simulink model "HybridCarModel"  (R2023a)
settings: Solver=VariableStepAuto  StartTime=0.0  StopTime=10.0  RelTol=1e-3
model workspace (MAT data in the model file):
  Aeff : Simulink.Parameter (value not decoded)
  Af : Simulink.Parameter (value not decoded)
  BattCapInit : Simulink.Parameter (value not decoded)
  BattChargeMax : Simulink.Parameter (value not decoded)
  BattTempBp : Simulink.Parameter (value not decoded)
  Bx : Simulink.Parameter (value not decoded)
  CapLUTBp : Simulink.Parameter (value not decoded)
  CapSOCBp : Simulink.Parameter (value not decoded)
  CatLightOffTime : Simulink.Parameter (value not decoded)
  Cd : Simulink.Parameter (value not decoded)
  Cl : Simulink.Parameter (value not decoded)
  Cpm : Simulink.Parameter (value not decoded)
  Cps : Simulink.Parameter (value not decoded)
  CrankSpeed : Simulink.Parameter (value not decoded)
  Cx : Simulink.Parameter (value not decoded)
  Dx : Simulink.Parameter (value not decoded)
  Em : Simulink.Parameter (value not decoded)
  EngRevLim : Simulink.Parameter (value not decoded)
  EngStopStartEnable : Simulink.Parameter (value not decoded)
  EngStopTime : Simulink.Parameter (value not decoded)
  Ex : Simulink.Parameter (value not decoded)
  FZMAX : Simulink.Parameter (value not decoded)
  FZMIN : Simulink.Parameter (value not decoded)
  Fc : Simulink.Parameter (value not decoded)
  FsbF : Simulink.Parameter (value not decoded)
  FsbR : Simulink.Parameter (value not decoded)
  FskF : Simulink.Parameter (value not decoded)
  FskR : Simulink.Parameter (value not decoded)
  G : Simulink.Parameter (value not decoded)
  G_o : Simulink.Parameter (value not decoded)
  Iyy : Simulink.Parameter (value not decoded)
  Iyy_Whl : Simulink.Parameter (value not decoded)
  J : Simulink.Parameter (value not decoded)
  J1 : Simulink.Parameter (value not decoded)
  J2 : Simulink.Parameter (value not decoded)
  Jd : Simulink.Parameter (value not decoded)
  Ji : Simulink.Parameter (value not decoded)
  Jin : Simulink.Parameter (value not decoded)
  Jin_Cltch : Simulink.Parameter (value not decoded)
  Jin_Cltch2 : Simulink.Parameter (value not decoded)
  Jout : Simulink.Parameter (value not decoded)
  Jout_Cltch : Simulink.Parameter (value not decoded)
  Jout_Cltch2 : Simulink.Parameter (value not decoded)
  Jt : Simulink.Parameter (value not decoded)
  Jw1 : Simulink.Parameter (value not decoded)
  Jw2 : Simulink.Parameter (value not decoded)
  K_c : Simulink.Parameter (value not decoded)
  Lrel : Simulink.Parameter (value not decoded)
  Mass : Simulink.Parameter (value not decoded)
  N : Simulink.Parameter (value not decoded)
  NCyl : Simulink.Parameter (value not decoded)
  NF : Simulink.Parameter (value not decoded)
  NR : Simulink.Parameter (value not decoded)
  N_P4 : Simulink.Parameter (value not decoded)
  N_idle : Simulink.Parameter (value not decoded)
  Ndiff : Simulink.Parameter (value not decoded)
  Ndiff_P4 : Simulink.Parameter (value not decoded)
  Ndisk : Simulink.Parameter (value not decoded)
  Ndisks : Simulink.Parameter (value not decoded)
  Np : Simulink.Parameter (value not decoded)
  Ns : Simulink.Parameter (value not decoded)
  Pabs : Simulink.Parameter (value not decoded)
  Plimit : Simulink.Parameter (value not decoded)
  Press : Simulink.Parameter (value not decoded)
  Pstd : Simulink.Parameter (value not decoded)
  RInt : Simulink.Parameter (value not decoded)
  Rair : Simulink.Parameter (value not decoded)
  Re : Simulink.Parameter (value not decoded)
  Reff : Simulink.Parameter (value not decoded)
  Reff_LSD : Simulink.Parameter (value not decoded)
  Rm : Simulink.Parameter (value not decoded)
  Sinj : Simulink.Parameter (value not decoded)
  T : Simulink.Parameter (value not decoded)
  T_eff_bp : Simulink.Parameter (value not decoded)
  T_t : Simulink.Parameter (value not decoded)
  Tc : Simulink.Parameter (value not decoded)
  Temp_bpts : Simulink.Parameter (value not decoded)
  Trq_bpts : Simulink.Parameter (value not decoded)
  Ts : Simulink.Parameter (value not decoded)
  Tstd : Simulink.Parameter (value not decoded)
  UNLOADED_RADIUS : Simulink.Parameter (value not decoded)
  VXLOW : Simulink.Parameter (value not decoded)
  Vd : Simulink.Parameter (value not decoded)
  Vinit : Simulink.Parameter (value not decoded)
  aMy : Simulink.Parameter (value not decoded)
  a_CG : Simulink.Parameter (value not decoded)
  afr_stoich : Simulink.Parameter (value not decoded)
  alphaMy : Simulink.Parameter (value not decoded)
  b : Simulink.Parameter (value not decoded)
  b1 : Simulink.Parameter (value not decoded)
  b1_g : Simulink.Parameter (value not decoded)
  b2 : Simulink.Parameter (value not decoded)
  b2_g : Simulink.Parameter (value not decoded)
  bMy : Simulink.Parameter (value not decoded)
  b_CG : Simulink.Parameter (value not decoded)
  b_J : Simulink.Parameter (value not decoded)
  bd : Simulink.Parameter (value not decoded)
  betaMy : Simulink.Parameter (value not decoded)
  bi : Simulink.Parameter (value not decoded)
  bin : Simulink.Parameter (value not decoded)
  bin_Cltch : Simulink.Parameter (value not decoded)
  bout : Simulink.Parameter (value not decoded)
  bout_Cltch : Simulink.Parameter (value not decoded)
  br : Simulink.Parameter (value not decoded)
  bt : Simulink.Parameter (value not decoded)
  bw1 : Simulink.Parameter (value not decoded)
  bw2 : Simulink.Parameter (value not decoded)
  cMy : Simulink.Parameter (value not decoded)
  calEngVar : object (value not decoded)
  disk_abore : Simulink.Parameter (value not decoded)
  domega_o : Simulink.Parameter (value not decoded)
  dw : Simulink.Parameter (value not decoded)
  dzdotsF : Simulink.Parameter (value not decoded)
  dzdotsR : Simulink.Parameter (value not decoded)
  dzsF : Simulink.Parameter (value not decoded)
  dzsR : Simulink.Parameter (value not decoded)
  eff : Simulink.Parameter (value not decoded)
  efficiency_table : Simulink.Parameter (value not decoded)
  eta : Simulink.Parameter (value not decoded)
  eta_diff : Simulink.Parameter (value not decoded)
  eta_tbl : Simulink.Parameter (value not decoded)
  f_cp_ld_bpt : Simulink.Parameter (value not decoded)
  f_cp_n_bpt : Simulink.Parameter (value not decoded)
  f_del_sa_bpt : Simulink.Parameter (value not decoded)
  f_ecp : Simulink.Parameter (value not decoded)
  f_egr_areapct_cmd : Simulink.Parameter (value not decoded)
  f_egr_areapct_nrmlzdflow_bpt : Simulink.Parameter (value not decoded)
  f_egr_areapct_pr_bpt : Simulink.Parameter (value not decoded)
  f_egr_max_stdflow : Simulink.Parameter (value not decoded)
  f_egr_stdflow : Simulink.Parameter (value not decoded)
  f_egr_stdflow_egrap_bpt : Simulink.Parameter (value not decoded)
  f_egr_stdflow_pr_bpt : Simulink.Parameter (value not decoded)
  f_egrpct_cmd : Simulink.Parameter (value not decoded)
  f_egrpct_ld_bpt : Simulink.Parameter (value not decoded)
  f_egrpct_n_bpt : Simulink.Parameter (value not decoded)
  f_fric_temp_bpt : Simulink.Parameter (value not decoded)
  f_fric_temp_mod : Simulink.Parameter (value not decoded)
  f_icp : Simulink.Parameter (value not decoded)
  f_intksys_stdflow_bpt : Simulink.Parameter (value not decoded)
  f_intksys_stdflow_pr : Simulink.Parameter (value not decoded)
  f_lamcmd : Simulink.Parameter (value not decoded)
  f_lamcmd_ld_bpt : Simulink.Parameter (value not decoded)
  f_lamcmd_n_bpt : Simulink.Parameter (value not decoded)
  f_lcmd : Simulink.Parameter (value not decoded)
  f_lcmd_n_bpt : Simulink.Parameter (value not decoded)
  f_lcmd_tq_bpt : Simulink.Parameter (value not decoded)
  f_m_lam : Simulink.Parameter (value not decoded)
  f_m_lam_bpt : Simulink.Parameter (value not decoded)
  f_m_sa : Simulink.Parameter (value not decoded)
  f_mdot_air_corr : Simulink.Parameter (value not decoded)
  f_mdot_air_corr_ld_bpt : Simulink.Parameter (value not decoded)
  f_mdot_air_n_bpt : Simulink.Parameter (value not decoded)
  f_mdot_intk : Simulink.Parameter (value not decoded)
  f_mdot_intk_ecp_bpt : Simulink.Parameter (value not decoded)
  f_mdot_trpd_bpt : Simulink.Parameter (value not decoded)
  f_nv : Simulink.Parameter (value not decoded)
  f_nv_n_bpt : Simulink.Parameter (value not decoded)
  f_nv_prs_bpt : Simulink.Parameter (value not decoded)
  f_sa : Simulink.Parameter (value not decoded)
  f_sa_ld_bpt : Simulink.Parameter (value not decoded)
  f_sa_n_bpt : Simulink.Parameter (value not decoded)
  f_sa_opt : Simulink.Parameter (value not decoded)
  f_startup_ect_bpt : Simulink.Parameter (value not decoded)
  f_startup_lambda_delta : Simulink.Parameter (value not decoded)
  f_startup_lambda_delta_timecnst : Simulink.Parameter (value not decoded)
  f_t_exh : Simulink.Parameter (value not decoded)
  f_t_exh_l_bpt : Simulink.Parameter (value not decoded)
  f_t_exh_n_bpt : Simulink.Parameter (value not decoded)
  f_tap : Simulink.Parameter (value not decoded)
  f_tap_ld_bpt : Simulink.Parameter (value not decoded)
  f_tap_n_bpt : Simulink.Parameter (value not decoded)
  f_tm_corr : Simulink.Parameter (value not decoded)
  f_tm_corr_n_bpt : Simulink.Parameter (value not decoded)
  f_tm_corr_nd_bpt : Simulink.Parameter (value not decoded)
  f_tpp : Simulink.Parameter (value not decoded)
  f_tpp_tap_bpt : Simulink.Parameter (value not decoded)
  f_tq_fric : Simulink.Parameter (value not decoded)
  f_tq_inr : Simulink.Parameter (value not decoded)
  f_tq_inr_l_bpt : Simulink.Parameter (value not decoded)
  f_tq_inr_n_bpt : Simulink.Parameter (value not decoded)
  f_tq_nl : Simulink.Parameter (value not decoded)
  f_tq_nl_l_bpt : Simulink.Parameter (value not decoded)
  f_tq_nl_n_bpt : Simulink.Parameter (value not decoded)
  f_tq_pump : Simulink.Parameter (value not decoded)
  f_vivc : Simulink.Parameter (value not decoded)
  f_vivc_icp_bpt : Simulink.Parameter (value not decoded)
  f_wap : Simulink.Parameter (value not decoded)
  f_wap_ld_bpt : Simulink.Parameter (value not decoded)
  f_wap_n_bpt : Simulink.Parameter (value not decoded)
  g : Simulink.Parameter (value not decoded)
  grEff : Simulink.Parameter (value not decoded)
  h : Simulink.Parameter (value not decoded)
  k : Simulink.Parameter (value not decoded)
  k1 : Simulink.Parameter (value not decoded)
  k2 : Simulink.Parameter (value not decoded)
  kappamax : Simulink.Parameter (value not decoded)
  lam_x : Simulink.Parameter (value not decoded)
  mu_kinetic : Simulink.Parameter (value not decoded)
  mu_static : Simulink.Parameter (value not decoded)
  muc : Simulink.Parameter (value not decoded)
  muk : Simulink.Parameter (value not decoded)
  mus : Simulink.Parameter (value not decoded)
  num_pads : Simulink.Parameter (value not decoded)
  omega1_c : Simulink.Parameter (value not decoded)
  omega2_c : Simulink.Parameter (value not decoded)
  omega_bpts : Simulink.Parameter (value not decoded)
  omega_c : Simulink.Parameter (value not decoded)
  omega_o : Simulink.Parameter (value not decoded)
  omega_o_J : Simulink.Parameter (value not decoded)
  omegai_o : Simulink.Parameter (value not decoded)
  omegain_o : Simulink.Parameter (value not decoded)
  omegal : Simulink.Parameter (value not decoded)
  omegao : Simulink.Parameter (value not decoded)
  omegaout_o : Simulink.Parameter (value not decoded)
  omegat_o : Simulink.Parameter (value not decoded)
  omegau : Simulink.Parameter (value not decoded)
  omegaw1o : Simulink.Parameter (value not decoded)
  omegaw2o : Simulink.Parameter (value not decoded)
  phi : Simulink.Parameter (value not decoded)
  philu : Simulink.Parameter (value not decoded)
  power_max : Simulink.Parameter (value not decoded)
  press : Simulink.Parameter (value not decoded)
  psi : Simulink.Parameter (value not decoded)
  q_o : Simulink.Parameter (value not decoded)
  tauC : Simulink.Parameter (value not decoded)
  tauC_1 : Simulink.Parameter (value not decoded)
  tauC_LSD : Simulink.Parameter (value not decoded)
  tauTC : Simulink.Parameter (value not decoded)
  tau_egr : Simulink.Parameter (value not decoded)
  tau_s : Simulink.Parameter (value not decoded)
  tc : Simulink.Parameter (value not decoded)
  theta_o : Simulink.Parameter (value not decoded)
  theta_o_Veh : Simulink.Parameter (value not decoded)
  torque_max : Simulink.Parameter (value not decoded)
  ts : Simulink.Parameter (value not decoded)
  w1_o : Simulink.Parameter (value not decoded)
  w_eff_bp : Simulink.Parameter (value not decoded)
  wc : Simulink.Parameter (value not decoded)
  win_o : Simulink.Parameter (value not decoded)
  wout_o : Simulink.Parameter (value not decoded)
  x_o : Simulink.Parameter (value not decoded)
  xdot_o : Simulink.Parameter (value not decoded)
  z_o : Simulink.Parameter (value not decoded)
  zdot_o : Simulink.Parameter (value not decoded)
  zeta : Simulink.Parameter (value not decoded)
symbols that are objects in the model workspace (value not decoded): b, b_CG, BattCapInit, BattChargeMax, CapLUTBp, Em, g, k, Mass, N, Ns, T, w_eff_bp
undefined symbols (not defined in the file or in its folder): Lock, up
libraries: autolibpowerinfoutils x5, autolibsharedcoupling x4, autolibshared x3, autolibutils x2, autolibshareddiff x2, autolibsharedmappedengines x1, autolibdcdc x1, autolibdatasheetbattery x1, autolibmappedmotor x1, autolibsharedtransfixedgear x1, autolibtrqconv x1
(part 3 of 3)

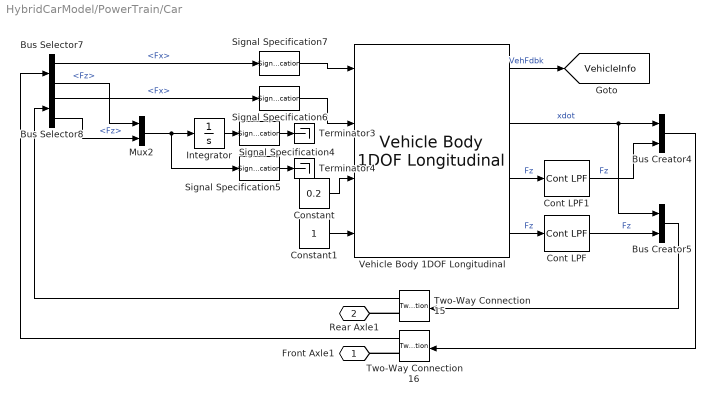
== system HybridCarModel/PowerTrain/Car ==
  Bus Creator4 : BusCreator  Inputs=2
  Bus Creator5 : BusCreator  Inputs=2
  Bus Selector7 : BusSelector  OutputSignals=Fx,Fz
  Bus Selector8 : BusSelector  OutputSignals=Fx,Fz
  Constant : Constant  Value=0.2
  Constant1 : Constant
  Cont LPF : autolibutils/Cont LPF  wc=wc  AbsoluteTolerance=auto  aMode=aMode
  Cont LPF1 : autolibutils/Cont LPF  wc=wc  AbsoluteTolerance=auto  aMode=aMode
  Integrator : Integrator
  Mux2 : Mux  Inputs=2
  Signal Specification4 : SignalSpecification  Unit=m
  Signal Specification5 : SignalSpecification  Unit=m/s
  Signal Specification6 : SignalSpecification  Unit=N
  Signal Specification7 : SignalSpecification  Unit=N
  Terminator3 : Terminator
  Terminator4 : Terminator
  Two-Way Connection15 : TwoWayConnection
  Two-Way Connection16 : TwoWayConnection
  Vehicle Body 1DOF Longitudinal : autolibshared/Vehicle Body 1DOF Longitudinal  VariantControl=SL  extFMode=off  extMMode=off  extTamb=off  wind3D=off  aMode=1  NF=NF  NR=NR  m=Mass  a=a_CG  b=b_CG  h=h  Cd=Cd  Cl=0  Cpm=0  Af=Af  x_o=x_o  xdot_o=xdot_o  Pabs=Pabs  T=T  g=g
      settings: LibrarySourceBlock=autolibvehdynlong/Vehicle Body 1DOF Longitudinal
  Front Axle1 : PMIOPort  Side=Left
  Rear Axle1 : PMIOPort  Port=2  Side=Left
  tag scope: VehicleInfo=global
  wires:
  Mux2/1 -> Signal Specification5/1, Integrator/1
  Vehicle Body 1DOF Longitudinal/2 -> Bus Creator4/1, Bus Creator5/1  "xdot"
  Bus Selector8/2 -> Mux2/2  "<Fz>"
  Bus Selector8/1 -> Signal Specification6/1  "<Fx>"
  Cont LPF1/1 -> Bus Creator4/2  "Fz"
  Bus Selector7/2 -> Mux2/1  "<Fz>"
  Signal Specification6/1 -> Vehicle Body 1DOF Longitudinal/2
  Two-Way Connection15/1 -> Bus Selector8/1
  Integrator/1 -> Signal Specification4/1
  Vehicle Body 1DOF Longitudinal/3 -> Cont LPF1/1  "Fz"
  Bus Creator5/1 -> Two-Way Connection15/1
  Signal Specification7/1 -> Vehicle Body 1DOF Longitudinal/1
  Vehicle Body 1DOF Longitudinal/1 -> [VehicleInfo]  "VehFdbk"
  Cont LPF/1 -> Bus Creator5/2  "Fz"
  Bus Creator4/1 -> Two-Way Connection16/1
  Bus Selector7/1 -> Signal Specification7/1  "<Fx>"
  Two-Way Connection16/1 -> Bus Selector7/1
  Signal Specification5/1 -> Terminator4/1
  Signal Specification4/1 -> Terminator3/1
  Vehicle Body 1DOF Longitudinal/4 -> Cont LPF/1  "Fz"
  Constant/1 -> Vehicle Body 1DOF Longitudinal/3
  Constant1/1 -> Vehicle Body 1DOF Longitudinal/4
  connections:
  Two-Way Connection16/RConn1 -- Front Axle1/RConn1
  Two-Way Connection15/RConn1 -- Rear Axle1/RConn1

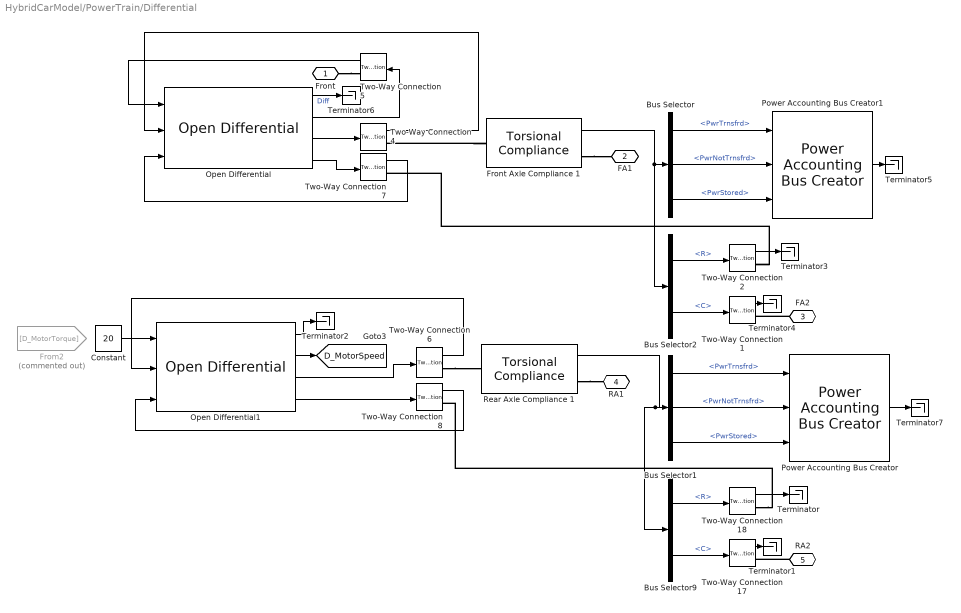
== system HybridCarModel/PowerTrain/Differential ==
  Bus Selector : BusSelector  OutputSignals=PwrInfo.PwrTrnsfrd,PwrInfo.PwrNotTrnsfrd,PwrInfo.PwrStored
  Bus Selector1 : BusSelector  OutputSignals=PwrInfo.PwrTrnsfrd,PwrInfo.PwrNotTrnsfrd,PwrInfo.PwrStored
  Bus Selector2 : BusSelector  OutputSignals=Trq.R,Trq.C
  Bus Selector9 : BusSelector  OutputSignals=Trq.R,Trq.C
  Constant : Constant  Value=20
  From2 : From  Commented=on  GotoTag=D_MotorTorque
  Front Axle Compliance 1 : autolibsharedcoupling/Torsional Compliance  port_config=Two-way connection  extInfo=on  k=k  b=b  theta_o=theta_o  domega_o=domega_o  omega_c=omega_c  blkID=0  aMode=1
  Open Differential : autolibshareddiff/Open Differential  DiffEffModelPopup=Constant  InterpMethod=Linear point-slope  extTamb=off  shaftSwitchMask=To the left of center-line  Ndiff=Ndiff  Jd=Jd  bd=bd  Jw1=Jw1  bw1=bw1  Jw2=Jw2  bw2=bw2  omegaw1o=omegaw1o  omegaw2o=omegaw2o  eta=eta_diff  eta_tbl=reshape([0.64 0.76 0.8 0.81 0.83 0.84 0.84 0.56 0.73 0.78 0.8 0.83 0.84 0.84 0.54 0.71 0.77 0.8 0.82 0.84 0.84 0.53 0.71 0.77 0.8 0.83 0.84 0.84 0.51 0.71 0.77 0.8 0.83 0.84 0.85 0.52 0.7 0.77 0.8 0.83 0.84 0.85 0.51 0.71 0.76 0.79 0.83 0.84 0.85 0.5 0.69 0.76 0.79 0.82 0.84 0.85 0.45 0.68 0.75 0.78 0.82 0.84 0.85 0.43 0.67 0.74 0.78 0.81 0.83 0.84 0.38 0.63 0.71 0.75 0.8 0.82 0.83 0.81 0.86 0.88 0.89 0.89 0.89 0.9 0.77 0.85 0.87 0.88 0.89 0.9 0.9 0.72 0.82 0.86 0.87 0.88 0.89 0.9 0.68 0.8 0.84 0.86 0.88 0.89 0.89 0.67 0.8 0.84 0.86 0.88 0.89 0.9 0.67 0.8 0.84 0.86 0.88 0.89 0.9 0.65 0.8 0.84 0.86 0.88 0.89 0.9 0.64 0.79 0.83 0.86 0.88 0.89 0.9 0.63 0.78 0.83 0.86 0.88 0.89 0.9 0.59 0.76 0.82 0.85 0.87 0.89 0.9 0.53 0.73 0.8 0.83 0.86 0.88 0.89], 7, 11, 2)  Trq_bpts=[25, 50, 75, 100, 150, 200, 250]  omega_bpts=[52.4 78.5 105 131 157 183 209 262 314 419 524]  Temp_bpts=[290 358]  Tamb=297.15  maxAbsSpd=5e3  aMode=1
      settings: LibrarySourceBlock=autolibdiff/Open Differential
  Open Differential1 : autolibshareddiff/Open Differential  DiffEffModelPopup=Constant  InterpMethod=Linear point-slope  extTamb=off  shaftSwitchMask=To the left of center-line  Ndiff=Ndiff_P4  Jd=Jd  bd=bd  Jw1=Jw1  bw1=bw1  Jw2=Jw2  bw2=bw2  omegaw1o=omegaw1o  omegaw2o=omegaw2o  eta=eta_diff  eta_tbl=reshape([0.64 0.76 0.8 0.81 0.83 0.84 0.84 0.56 0.73 0.78 0.8 0.83 0.84 0.84 0.54 0.71 0.77 0.8 0.82 0.84 0.84 0.53 0.71 0.77 0.8 0.83 0.84 0.84 0.51 0.71 0.77 0.8 0.83 0.84 0.85 0.52 0.7 0.77 0.8 0.83 0.84 0.85 0.51 0.71 0.76 0.79 0.83 0.84 0.85 0.5 0.69 0.76 0.79 0.82 0.84 0.85 0.45 0.68 0.75 0.78 0.82 0.84 0.85 0.43 0.67 0.74 0.78 0.81 0.83 0.84 0.38 0.63 0.71 0.75 0.8 0.82 0.83 0.81 0.86 0.88 0.89 0.89 0.89 0.9 0.77 0.85 0.87 0.88 0.89 0.9 0.9 0.72 0.82 0.86 0.87 0.88 0.89 0.9 0.68 0.8 0.84 0.86 0.88 0.89 0.89 0.67 0.8 0.84 0.86 0.88 0.89 0.9 0.67 0.8 0.84 0.86 0.88 0.89 0.9 0.65 0.8 0.84 0.86 0.88 0.89 0.9 0.64 0.79 0.83 0.86 0.88 0.89 0.9 0.63 0.78 0.83 0.86 0.88 0.89 0.9 0.59 0.76 0.82 0.85 0.87 0.89 0.9 0.53 0.73 0.8 0.83 0.86 0.88 0.89], 7, 11, 2)  Trq_bpts=[25, 50, 75, 100, 150, 200, 250]  omega_bpts=[52.4 78.5 105 131 157 183 209 262 314 419 524]  Temp_bpts=[290 358]  Tamb=297.15  maxAbsSpd=5e3  aMode=1
      settings: LibrarySourceBlock=autolibdiff/Open Differential
  Power Accounting Bus Creator : autolibpowerinfoutils/Power Accounting Bus Creator  AssctBlkSelPopup=Parent  RefBlkName='libraryname/blkname'  PwrTrnsfrdCheckBox=on  PwrNotTrnsfrdCheckBox=on  PwrStoredCheckBox=on  aMode=aMode
  Power Accounting Bus Creator1 : autolibpowerinfoutils/Power Accounting Bus Creator  AssctBlkSelPopup=Parent  RefBlkName='libraryname/blkname'  PwrTrnsfrdCheckBox=on  PwrNotTrnsfrdCheckBox=on  PwrStoredCheckBox=on  aMode=aMode
  Rear Axle Compliance 1 : autolibsharedcoupling/Torsional Compliance  port_config=Two-way connection  extInfo=on  k=k  b=b  theta_o=theta_o  domega_o=domega_o  omega_c=omega_c  blkID=0  aMode=1
  Terminator{,1..7} (8 alike) : Terminator
  Two-Way Connection{1..2,4..8,17..18} (9 alike) : TwoWayConnection
  Front : PMIOPort  Side=Left
  FA1 : PMIOPort  Port=2  Side=Right
  FA2 : PMIOPort  Port=3  Side=Right
  RA1 : PMIOPort  Port=4  Side=Right
  RA2 : PMIOPort  Port=5  Side=Right
  tag scope: D_MotorSpeed=global
  wires:
  Open Differential1/2 -> [D_MotorSpeed]
  Rear Axle Compliance 1/1 -> Bus Selector9/1, Bus Selector1/1
  Bus Selector9/1 -> Two-Way Connection18/1  "<R>"
  Two-Way Connection5/1 -> Open Differential/1
  Open Differential1/3 -> Two-Way Connection6/1
  Two-Way Connection4/1 -> Open Differential/2
  Two-Way Connection8/1 -> Open Differential1/3
  Open Differential1/1 -> Terminator2/1
  Open Differential/1 -> Terminator6/1  "Diff"
  Two-Way Connection17/1 -> Terminator1/1
  Two-Way Connection6/1 -> Open Differential1/2
  Two-Way Connection7/1 -> Open Differential/3
  Bus Selector1/2 -> Power Accounting Bus Creator/2  "<PwrNotTrnsfrd>"
  Open Differential/3 -> Two-Way Connection4/1
  Open Differential/4 -> Two-Way Connection7/1
  Open Differential/2 -> Two-Way Connection5/1
  Two-Way Connection18/1 -> Terminator/1
  Open Differential1/4 -> Two-Way Connection8/1
  Bus Selector9/2 -> Two-Way Connection17/1  "<C>"
  Power Accounting Bus Creator/1 -> Terminator7/1
  Bus Selector1/3 -> Power Accounting Bus Creator/3  "<PwrStored>"
  Bus Selector1/1 -> Power Accounting Bus Creator/1  "<PwrTrnsfrd>"
  Power Accounting Bus Creator1/1 -> Terminator5/1
  Bus Selector2/1 -> Two-Way Connection2/1  "<R>"
  Two-Way Connection1/1 -> Terminator4/1
  Two-Way Connection2/1 -> Terminator3/1
  Bus Selector2/2 -> Two-Way Connection1/1  "<C>"
  Front Axle Compliance 1/1 -> Bus Selector2/1, Bus Selector/1
  Bus Selector/1 -> Power Accounting Bus Creator1/1  "<PwrTrnsfrd>"
  Bus Selector/3 -> Power Accounting Bus Creator1/3  "<PwrStored>"
  Bus Selector/2 -> Power Accounting Bus Creator1/2  "<PwrNotTrnsfrd>"
  Constant/1 -> Open Differential1/1
  connections:
  Front/RConn1 -- Two-Way Connection5/RConn1
  FA2/RConn1 -- Two-Way Connection1/RConn1
  Two-Way Connection2/RConn1 -- Two-Way Connection7/RConn1
  Front Axle Compliance 1/LConn1 -- Two-Way Connection4/RConn1
  Front Axle Compliance 1/RConn1 -- FA1/RConn1
  Rear Axle Compliance 1/RConn1 -- RA1/RConn1
  Two-Way Connection6/RConn1 -- Rear Axle Compliance 1/LConn1
  RA2/RConn1 -- Two-Way Connection17/RConn1
  Two-Way Connection18/RConn1 -- Two-Way Connection8/RConn1

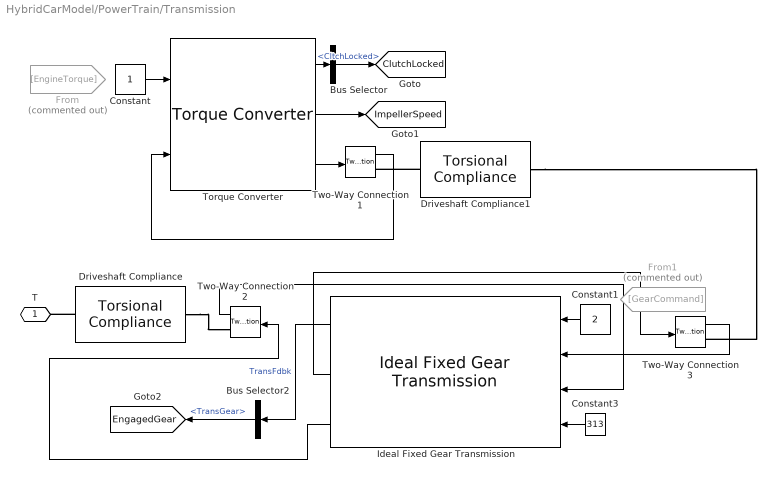
== system HybridCarModel/PowerTrain/Transmission ==
  Bus Selector : BusSelector  OutputSignals=Cltch.CltchLocked
  Bus Selector2 : BusSelector  OutputSignals=Trans.TransGear
  Constant : Constant
  Constant1 : Constant  Value=2
  Constant3 : Constant  Value=313
  Driveshaft Compliance : autolibsharedcoupling/Torsional Compliance  port_config=Two-way connection  extInfo=off  k=k  b=b  theta_o=theta_o  domega_o=domega_o  omega_c=omega_c  blkID=0  aMode=1
  Driveshaft Compliance1 : autolibsharedcoupling/Torsional Compliance  port_config=Two-way connection  extInfo=off  k=k  b=b  theta_o=theta_o  domega_o=domega_o  omega_c=omega_c  blkID=0  aMode=1
  From : From  Commented=on  GotoTag=EngineTorque
  From1 : From  Commented=on  GotoTag=GearCommand
  Ideal Fixed Gear Transmission : autolibsharedtransfixedgear/Ideal Fixed Gear Transmission  VariantControl=0  TransEffModelPopup=Gear, input torque, input speed, and temperature  gearInterp=Linear point-slope  G=G  Trq_bpts=Trq_bpts  omega_bpts=omega_bpts  Temp_bpts=Temp_bpts  N=N  Jout=Jout  bout=bout  eta=eta  eta_tbl=eta_tbl  G_o=0  omega_o=omega_o  omegaN_o=0  tau_s=tau_s  maxAbsSpd=5e3  aMode=1
      settings: LibrarySourceBlock=autolibtrans/Ideal Fixed Gear Transmission
  Torque Converter : autolibtrqconv/Torque Converter  TCType=Lock-up  port_config=Simulink  Ji=Ji  bi=bi  Jt=Jt  bt=bt  omegai_o=omegai_o  omegat_o=omegat_o  phi=phi  KType=Input speed / sqrt(input torque)  psi=psi  zeta=zeta  tauTC=tauTC  InterpMethod=Linear  Reff=Reff  mus=mus  muk=muk  ClutchLocked=off  philu=philu  omegal=omegal  omegau=omegau  K_c=K_c  tauC=tauC  maxAbsSpd=5e3  tau_dl=3000
      settings: AttributesFormatString="Lock-up type:  %<TCType>"
  Two-Way Connection1 : TwoWayConnection
  Two-Way Connection2 : TwoWayConnection
  Two-Way Connection3 : TwoWayConnection
  T : PMIOPort  Side=Right
  tag scope: ClutchLocked=global, EngagedGear=global, ImpellerSpeed=global
  wires:
  Ideal Fixed Gear Transmission/3 -> Two-Way Connection2/1
  Bus Selector/1 -> [ClutchLocked]  "<CltchLocked>"
  Ideal Fixed Gear Transmission/2 -> Two-Way Connection3/1
  Two-Way Connection3/1 -> Ideal Fixed Gear Transmission/2
  Ideal Fixed Gear Transmission/1 -> Bus Selector2/1  "TransFdbk"
  Torque Converter/3 -> Two-Way Connection1/1
  Two-Way Connection2/1 -> Ideal Fixed Gear Transmission/3
  Two-Way Connection1/1 -> Torque Converter/2
  Torque Converter/2 -> [ImpellerSpeed]
  Constant3/1 -> Ideal Fixed Gear Transmission/4
  Bus Selector2/1 -> [EngagedGear]  "<TransGear>"
  Torque Converter/1 -> Bus Selector/1
  Constant/1 -> Torque Converter/1
  Constant1/1 -> Ideal Fixed Gear Transmission/1
  connections:
  Driveshaft Compliance/LConn1 -- Two-Way Connection2/RConn1
  Driveshaft Compliance/RConn1 -- T/RConn1
  Driveshaft Compliance1/LConn1 -- Two-Way Connection1/RConn1
  Driveshaft Compliance1/RConn1 -- Two-Way Connection3/RConn1
